simulink model "lab5_ECU2"  (R2018a)
settings: Solver=FixedStepDiscrete  StartTime=0.0  StopTime=10.0  RelTol=1e-3
undefined symbols (not defined in the file or in its folder): ECU565, motohawk_build_version, motohawk_trunc_name, motohawk_vardec_path
libraries: MotoHawk_lib x12, motohawk_examples_lib x1, MotoHawk_Protocols_lib x1
settings Model: MotoHawkModelGUID=7117BFC8-B046-410F-A68B-2915BCBA8DCA  MotoHawkModelOpenTime=2019 3 19 13 38 14.751  MotoHawkBuildVersion=000  MotoHawkBuildStats=struct('TotalFLASH',{0},'TotalEEPROM',{0},'TotalRAM',{0},'AppFLASH',{0},'AppEEPROM',{0},'AppRAM',{0},'HeapRAM',{0},'BuildSuccessCount',{0},'BuildErrorCount',{0})  MotoHawkBuildDirectory=C:\Users\dhruv\OneDrive\Desktop\MEEM 5750\Lab\Lab 5\lab5_ECU2_Build  MotoHawkBuildInfo=struct('refmodel',{0},'model_name',{'lab5_ECU2'},'motohawk_version',{'2018a_sp2.2221'},'motohawk_component_version',{'0.0.8'},'motohawk_refmdl_version',{'0.0.1'},'matlab_version',{'9.4.0'},'build_version',{'000'},'module_type',{'ECU565-128'},'layout_type',{'DEV'},'enable_build',{1},'processor_family',{'PPC'},'processor_type',{'MPC565'},'toolchain_vendor',{'gcc-powerpc-eabi'},'toolchain_version',{'4.6.0'},'component',{0},'archive_file',{'PCM128.a'},'fptype',{0},'flash_size',{1048576},'ee_size',{8192},'ram_size',{36864},'decram_size',{4096},'eri_table0_rev',{9},'max_eri_table_size',{65535},'fgnd_base_period_ms',{5},'bgnd_base_period_ms',{50},'build_dir',{'C:\Users\dhruv\OneDrive\Desktop\MEEM 5750\Lab\Lab 5\lab5_ECU2_Build'},'dll_name',{'lab5_ECU2_000'},'srz_name',{'lab5_ECU2_000'},'fgnd_stack_size',{3072},'fgnd_angle_stack_size',{0},'bgnd_stack_size',{2048},'idle_stack_size',{1024},'irq_stack_size',{1536},'irq_stack_margin',{153},'heap_size',{4096},'heap_margin',{409},'app_int_stack_size',{1024},'shutdown_stack_size',{1024},'use_target_os_config',{0},'num_cores_in_use',{1},'target_os',{'Classic ControlCore'},'install_dll_dir',{'C:\ECUFiles\TDBDLL'},'install_srz_dir',{'C:\ECUFiles\Programs'},'mingw_dir',{'C:\Program Files (x86)\Woodward\DevelopmentTools\Toolchains\GCC\win64-pe\4_7_1'},'motohawk_dir',{'C:\Program Files (x86)\Woodward\MCS\MotoHawk\2018a_sp2.2221'},'toolchain_dir',{'C:\Program Files (x86)\Woodward\DevelopmentTools\Toolchains\GCC\powerpc-eabi\4_6_0'},'matlab_root',{'C:\Program Files\MATLAB\R2018a'},'model_guid',{'7117BFC8-B046-410F-A68B-2915BCBA8DCA'},'build_guid',{[]},'token_guid',{'no token'})  MotoHawkCANInfo=struct('DefnArr',{struct('res_name',{'CAN_1'},'text_resource',{'CAN1'},'IsSupportedMethodArr',{logical([1;0;0;0;0;0;0;0;0;0;0])})})  MotoHawkModelSavedName=lab5_ECU2  MotoHawkModelElapsedTime=39104.721  Creator=dhruv  LastModifiedBy=dhruv
settings ConfigSet: Description="This Simulink Configuration Set is preconfigured  for the MotoHawk target \"ECU565-128\"."
settings OptimizationCC: DefaultParameterBehavior=Inlined  InlineInvariantSignals=on  EnhancedBackFolding=on  PassReuseOutputArgsAs=Individual arguments  InitFltsAndDblsToZero=on  NoFixptDivByZeroProtection=on  EfficientFloat2IntCast=on  LifeSpan=1  OptimizeBlockOrder=speed  DifferentSizesBufferReuse=on  OptimizationCustomize=off
settings DebuggingCC: InheritedTsInSrcMsg=none  TasksWithSamePriorityMsg=none  ParameterTunabilityLossMsg=error  ModelReferenceIOMismatchMessage=warning
settings HardwareCC: ProdBitPerPointer=32  ProdBitPerSizeT=32  ProdBitPerPtrDiffT=32  ProdLargestAtomicInteger=Integer  ProdIntDivRoundTo=Undefined  ProdEndianess=BigEndian  ProdWordSize=32  ProdHWDeviceType=Specified
settings ModelReferenceCC: UpdateModelReferenceTargets=IfOutOfDate  CheckModelReferenceTargetMessage=warning  ModelReferenceNumInstancesAllowed=Single
settings SFSimCC: MATLABDynamicMemAlloc=off
settings RTWCC: SystemTargetFile=motohawk_ert_rtw.tlc  MakeCommand=make_rtw_motohawk  TemplateMakefile=motohawk_ert_rtw.tmf  Description=MotoHawk(tm) Rapid Prototyping  GenerateReport=on  IncludeHyperlinkInReport=on  LaunchReport=on  GenerateTraceInfo=on  GenerateTraceReport=on  GenerateTraceReportSl=on  GenerateTraceReportSf=on  GenerateTraceReportEml=on
settings CodeAppCC: ForceParamTrailComments=on  IgnoreCustomStorageClasses=off  MaxIdLength=100  OperatorAnnotations=on  SimulinkDataObjDesc=on  SFDataObjDesc=on  CustomSymbolStrType=$N$R$M  CustomSymbolStrField=$H$N$M  InsertBlockDesc=on  InternalIdentifier=Classic
settings STFCustomTargetCC: TargetLangStandard=C99 (ISO)  MultiwordTypeDef=User defined  MultiwordLength=256  IncludeMdlTerminateFcn=off  GeneratePreprocessorConditionals=Disable all  CombineOutputUpdateFcns=on  SuppressErrorStatus=on  ERTCustomFileBanners=on  SupportContinuousTime=off  SupportNonInlinedSFcns=off  RemoveResetFunc=on  MATLABClassNameForMDSCustomization=Simulink.SoftwareTarget.ERTCustomization  GRTInterface=off  SystemTargetFile=motohawk_ert_rtw.tlc
settings ERTTargetCC: TargetLangStandard=C99 (ISO)  MultiwordTypeDef=User defined  MultiwordLength=0  ParMdlRefBuildCompliant=off  CompOptLevelCompliant=off  ConcurrentExecutionCompliant=off  IncludeMdlTerminateFcn=off  GeneratePreprocessorConditionals=Disable all  SuppressErrorStatus=on  ModelStepFunctionPrototypeControlCompliant=off  CPPClassGenCompliant=off  UseToolchainInfoCompliant=off  InlinedParameterPlacement=NonHierarchical  ERTCustomFileTemplate=example_file_process.tlc

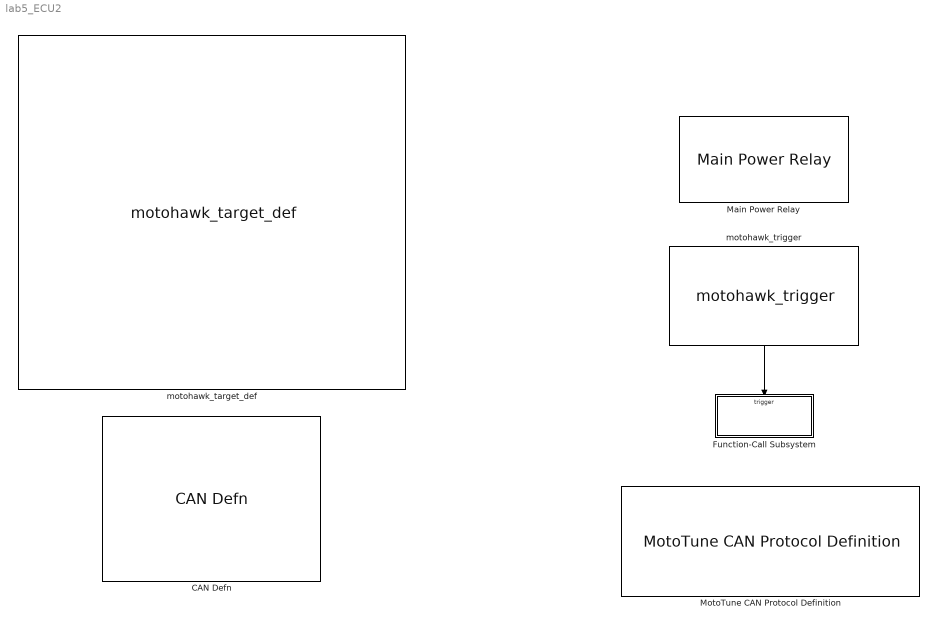
== system lab5_ECU2 ==
  CAN Defn : MotoHawk_lib/CAN Blocks/CAN Defn  Priority=-100  res_name='CAN_1'  text_resource=CAN1  target=ECU565-128  bit_time_src=Default  update_without_reboot=off  btime=250000  baud_rate_src=Constant  baud_rate=uint32(250000)  baud_rate_data_store_name='CAN1_BaudRate'  sample_point_tq_src=Constant  sample_point_tq=6  sample_point_tq_data_store_name='SamplePoint_TQ'  total_tq_src=Constant  total_tq=8  total_tq_data_store_name='Total_TQ'  synch_jw_src=Constant  synch_jw=1  synch_jw_data_store_name='SynchJumpWidth'  tx_queue_size=16  rx_queue_size=16
      settings: SourceProductName=MotoHawk
  Function-Call Subsystem : Subsystem  TreatAsAtomicUnit=on
  Main Power Relay : motohawk_examples_lib/Main Power Relay Blocks/Main Power Relay  on_delay_count=2  off_delay_count=5  ecup_threshold=100  group='System | Main Power Relay'
      settings: SourceProductName=MotoHawk
  MotoTune CAN Protocol Definition : MotoHawk_Protocols_lib/MotoTune Blocks/MotoTune CAN Protocol Definition  Priority=-100  nam='MotoTuneHandler'  ref_name='CAN_1'  city_id_src=Constant  city_id=hex2dec('0C')  city_id_data_store_name='CityID'
      settings: SourceProductName=MotoHawk
  motohawk_target_def : MotoHawk_lib/motohawk_target_def  Priority=-65535  target=ECU565-128  layout=DEV  fptype=single (32 bits)  use_target_os_config=off  target_os=ControlCore  default_target_os=Classic ControlCore  fgnd_stack_size=3*1024  fgnd_angle_stack_size=0  bgnd_stack_size=2*1024  idle_stack_size=1024  irq_stack_size=1536  app_int_stack_size=1024  shutdown_stack_size=1024  heap_size=4*1024  show_margins=off  fgnd_stack_margin=(3*1024) * 0.1  fgnd_angle_stack_margin=0  bgnd_stack_margin=(2*1024) * 0.1  idle_stack_margin=(1024) * 0.1  irq_stack_margin=(1536) * 0.1  app_int_stack_margin=(1024) * 0.1  shutdown_stack_margin=(1024) * 0.1  heap_margin=(4*1024) * 0.1  comp_name=bdroot  comp_img='KVASER_CAN_USB.jpg'  comp_security=No Encryption  comp_build_pass='mhbuild'  comp_sim_pass='mhsim'  comp_multi=off  show_filenames=off  dll_name=motohawk_trunc_name(bdroot, ['_' motohawk_build_version], 50)  srz_name=motohawk_trunc_name(bdroot, ['_' motohawk_build_version], 50)  build_dir='.'  comp_dir='.'
      settings: SourceProductName=MotoHawk
  motohawk_trigger : MotoHawk_lib/Trigger Blocks/motohawk_trigger  Tag=Trigger  Priority=0  trig_name=[]  trigger=FGND_RTI_PERIODIC  priority_order=0  inherited=off  run_disabled=off  override_app_monitor=off  target=ECU565_128
      settings: SourceProductName=MotoHawk
  wires:
  motohawk_trigger/1 -> Function-Call Subsystem/Trigger

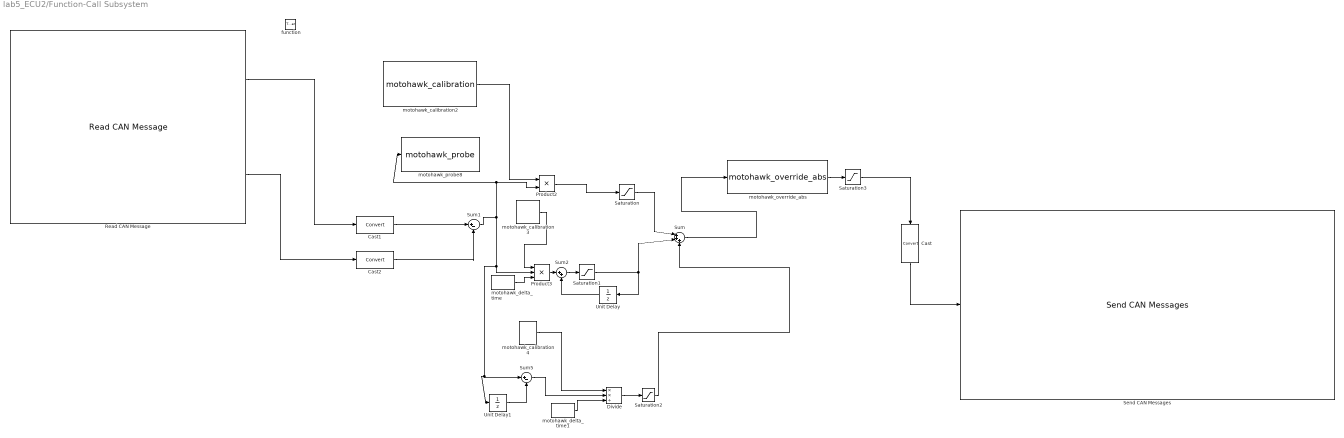
== system lab5_ECU2/Function-Call Subsystem ==
  function : TriggerPort  TriggerType=function-call  VariantControl=Variant
  Cast : DataTypeConversion
  Cast1 : DataTypeConversion
  Cast2 : DataTypeConversion
  Divide : Product  Inputs=**/
  Product2 : Product
  Product3 : Product  Inputs=3
  Read CAN Message : MotoHawk_lib/CAN Blocks/Read CAN Message  nam='CAN_1'  bus=-2  msg=etc_can_template  queue=1  slot=''  valid=off  stale=off  labelwires=off
      settings: SourceProductName=MotoHawk
  Saturation : Saturate
  Saturation1 : Saturate
  Saturation2 : Saturate
  Saturation3 : Saturate  UpperLimit=0.35  LowerLimit=0
  Send CAN Messages : MotoHawk_lib/CAN Blocks/Send CAN Messages  bus=-2  nam='CAN_1'  msgl=pwmtemplate  pace=5  labelwires=off
      settings: SourceProductName=MotoHawk
  Sum : Sum  Inputs=|+++
  Sum1 : Sum  Inputs=|+-
  Sum2 : Sum  Inputs=|++
  Sum5 : Sum  Inputs=|+-
  Unit Delay : UnitDelay  SampleTime=-1
  Unit Delay1 : UnitDelay  SampleTime=-1
  motohawk_calibration2 : MotoHawk_lib/Calibration & Probing Blocks/motohawk_calibration  nam='Kp'  val=0  storage=Calibration  show_more=off  name_source=Use Parameter  data_type=Inherit from 'Default Value'  read_level=1  write_level=1  ovr_cals=on  view_as=Number  enum_struct={'Disabled', 'Enabled'}  vector_style=Wide Row  use_help_units=off  help=''  units=''  use_header_enum=off  row_header_enum={}  col_header_enum={}  use_min_max=off  min_val=-inf  max_val=inf  use_precision=off  precision=''  gain=1  offset=0  exp=1  use_mototune_group=off  mototune_group=motohawk_vardec_path(gcb)  data_stores=motohawk_sfun_calibration_data_stores
      settings: SourceProductName=MotoHawk
  motohawk_calibration3 : MotoHawk_lib/Calibration & Probing Blocks/motohawk_calibration  nam='KI'  val=0  storage=Calibration  show_more=off  name_source=Use Parameter  data_type=Inherit from 'Default Value'  read_level=1  write_level=1  ovr_cals=on  view_as=Number  enum_struct={'Disabled', 'Enabled'}  vector_style=Wide Row  use_help_units=off  help=''  units=''  use_header_enum=off  row_header_enum={}  col_header_enum={}  use_min_max=off  min_val=-inf  max_val=inf  use_precision=off  precision=''  gain=1  offset=0  exp=1  use_mototune_group=off  mototune_group=motohawk_vardec_path(gcb)  data_stores=motohawk_sfun_calibration_data_stores
      settings: SourceProductName=MotoHawk
  motohawk_calibration4 : MotoHawk_lib/Calibration & Probing Blocks/motohawk_calibration  nam='Kd'  val=0  storage=Calibration  show_more=off  name_source=Use Parameter  data_type=Inherit from 'Default Value'  read_level=1  write_level=1  ovr_cals=on  view_as=Number  enum_struct={'Disabled', 'Enabled'}  vector_style=Wide Row  use_help_units=off  help=''  units=''  use_header_enum=off  row_header_enum={}  col_header_enum={}  use_min_max=off  min_val=-inf  max_val=inf  use_precision=off  precision=''  gain=1  offset=0  exp=1  use_mototune_group=off  mototune_group=motohawk_vardec_path(gcb)  data_stores=motohawk_sfun_calibration_data_stores
      settings: SourceProductName=MotoHawk
  motohawk_delta_time : MotoHawk_lib/Extra Development Blocks/motohawk_delta_time  samp_time=-1  init_val=0  mode=Seconds (double)
      settings: SourceProductName=MotoHawk
  motohawk_delta_time1 : MotoHawk_lib/Extra Development Blocks/motohawk_delta_time  samp_time=-1  init_val=0  mode=Seconds (double)
      settings: SourceProductName=MotoHawk
  motohawk_override_abs : MotoHawk_lib/Calibration & Probing Blocks/motohawk_override_abs  parent_name='Override_Absolute_PWM'  parent_val=0  show_more=off  name_source=Use Parameter  parent_read_level=1  parent_override_level=1  view_as=Number  enum_struct={'Disabled', 'Enabled'}  use_help_units=off  parent_help=''  parent_units=''  use_min_max=off  parent_min=-inf  parent_max=inf  use_precision=off  parent_precision=''  parent_gain=1  parent_offset=0  parent_exp=1  use_mototune_group=off  parent_group=motohawk_vardec_path(gcb)
      settings: SourceProductName=MotoHawk
  motohawk_probe8 : MotoHawk_lib/Calibration & Probing Blocks/motohawk_probe  nam='Error_input'  show_more=off  name_source=Use Parameter  read_level=1  view_as=Number  enum_struct={'Disabled', 'Enabled'}  vector_style=Wide Row  use_help_units=off  help=''  units=''  use_header_enum=off  row_header_enum={}  col_header_enum={}  use_min_max=off  min_val=-inf  max_val=inf  use_precision=off  precision=''  gain=1  offset=0  exp=1  use_mototune_group=off  mototune_group=motohawk_vardec_path(gcb)
      settings: SourceProductName=MotoHawk
  wires:
  motohawk_delta_time1/1 -> Divide/3
  motohawk_calibration2/1 -> Product2/1
  Sum/1 -> motohawk_override_abs/1
  motohawk_override_abs/1 -> Saturation3/1
  motohawk_calibration3/1 -> Product3/1
  Divide/1 -> Saturation2/1
  Sum2/1 -> Saturation1/1
  Read CAN Message/2 -> Cast2/1
  motohawk_calibration4/1 -> Divide/1
  Saturation2/1 -> Sum/3
  Sum1/1 -> Product2/2, motohawk_probe8/1, Unit Delay1/1, Sum5/1, Product3/2
  Product3/1 -> Sum2/1
  Sum5/1 -> Divide/2
  motohawk_delta_time/1 -> Product3/3
  Saturation/1 -> Sum/1
  Unit Delay1/1 -> Sum5/2
  Unit Delay/1 -> Sum2/2
  Product2/1 -> Saturation/1
  Saturation1/1 -> Unit Delay/1, Sum/2
  Read CAN Message/1 -> Cast1/1
  Saturation3/1 -> Cast/1
  Cast/1 -> Send CAN Messages/1
  Cast1/1 -> Sum1/1
  Cast2/1 -> Sum1/2
